simulink model "block_lms"  (Simulink 7.8)
settings: Solver=ode45  StartTime=0.0  StopTime=0.05  RelTol=1e-3
values from neighbouring files (symbols this model uses):
  h = firpm(64,f,m)    [CFIR_1.m]    (also in adapt_filter1.m = adaptfilt.lms(ni,mu); adapt_filter2.m = adaptfilt.blms(ni,mu,1,36); adaptiv_2.m = [1 2 3 4 5 6 7 8 9 10]; adaptiv_3.m = [1 2 3 4 5 6 7 8 9 10])
  hmusik = fir1(nf-1, 0.4)    [block_lms_.m]
  hr = 0.8.^(0:nf-1)    [block_lms_.m]
  M = 2    [CFIR_1.m]    (also in block_lms_.m = 16; cic_dezim1.m = ',num2str(M),'; cic_dezim1_.m = ',num2str(M),     '; cic_dezim2.m = ',num2str(M),')
  Ts = 1/fs    (= 6.25e-05)    [G722_1.m]    (also in adaptiv_2.m = 0.001; adaptiv_3.m = 0.001; adaptiv_4.m = 0.001; adaptiv_5.m = 0.001)
undefined symbols (not defined in the file or in its folder): get, stoerung
libraries: dspsigops x1, dspadpt3 x1, dspsrcs4 x1, dspsnks4 x1
settings Model: Creator=svenhoffmann  LastModifiedBy=josef  ExtModeAutoUpdateStatusClock=off
settings DataIOCC: SignalLoggingName=sigsOut
settings DebuggingCC: SaveWithParameterizedLinksMsg=none  SignalResolutionControl=TryResolveAllWithWarning  SolverPrmCheckMsg=none  MultiTaskDSMMsg=warning  MultiTaskCondExecSysMsg=none  StrictBusMsg=None
settings HardwareCC: TargetUnknown=on
settings RTWCC: IncludeERTFirstTime=on

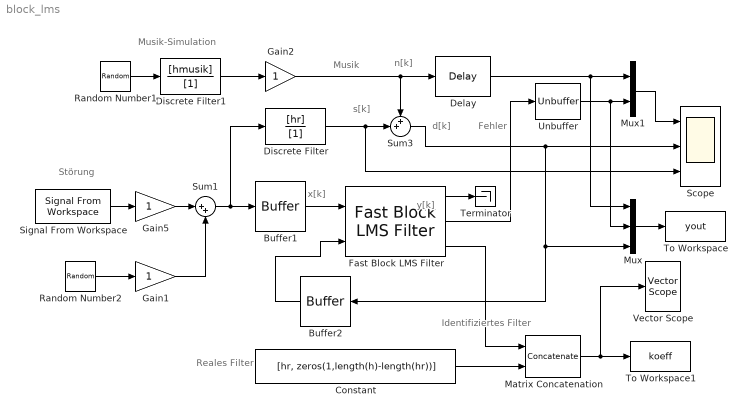
== system block_lms ==
  note: Musik
  note: Störung
  note: Musik-Simulation
  note: Fehler
  note: s[k]
  note: n[k]
  note: d[k]
  note: y[k]
  note: x[k]
  note: Reales Filter
  note: Identifiziertes Filter
  Buffer1 : Buffer  N=M
  Buffer2 : Buffer  N=M
  Constant : Constant  Value=[hr, zeros(1,length(h)-length(hr))]
  Delay : dspsigops/Delay  InputProcessing=Inherited (this choice will be removed - see release notes)  dly_unit=Samples  delay=M  ic_detail=off  dif_ic_for_ch=off  dif_ic_for_dly=off  ic=0  reset_popup=None
  Discrete Filter : DiscreteFilter  Numerator=[hr]  Denominator=[1]
  Discrete Filter1 : DiscreteFilter  Numerator=[hmusik]  Denominator=[1]  SampleTime=Ts
  Fast Block LMS Filter : dspadpt3/Fast Block LMS Filter  algo=Fast Block LMS  L=M  N=M  stepflag=Dialog  mu=0.002  leakage=1.0  addnparflag=off  ic=0  Adapt=off  resetflag=None  weights=on
  Gain1 : Gain  SaturateOnIntegerOverflow=on  OutDataTypeStr=Inherit: Same as input  ParamDataTypeStr=Inherit: Same as input
  Gain2 : Gain  SaturateOnIntegerOverflow=on  OutDataTypeStr=Inherit: Same as input  ParamDataTypeStr=Inherit: Same as input
  Gain5 : Gain  SaturateOnIntegerOverflow=on  OutDataTypeStr=Inherit: Same as input  ParamDataTypeStr=Inherit: Same as input
  Matrix Concatenation : Concatenate  Mode=Multidimensional array  ConcatenateDimension=2
  Mux : Mux  Inputs=3
  Mux1 : Mux  Inputs=2
  Random Number1 : RandomNumber  Seed=1739  SampleTime=Ts
  Random Number2 : RandomNumber  SampleTime=Ts
  Scope : Scope  NumInputPorts=3
      settings: YMin=-2.25~-2.25~-1  YMax=2.25~2.25~0.8
  Signal From Workspace : dspsrcs4/Signal From Workspace  X=stoerung(:,1)  Ts=Ts  nsamps=1  OutputAfterFinalValue=Setting to zero  ignoreOrWarnInputAndFrameLengths=off
  Sum1 : Sum  Inputs=|++  SaturateOnIntegerOverflow=on
  Sum3 : Sum  Inputs=++|  SaturateOnIntegerOverflow=on
  Terminator : Terminator
  To Workspace : ToWorkspace  VariableName=yout  SampleTime=-1  SaveFormat=Structure With Time
  To Workspace1 : ToWorkspace  VariableName=koeff  SampleTime=-1  SaveFormat=Structure
      settings: Decimation=100
  Unbuffer : Unbuffer
  Vector Scope : dspsnks4/Vector Scope  ScopeProperties=off  Domain=Time  HorizSpan=1  DisplayProperties=off  AxisGrid=on  Memory=off  FrameNumber=on  AxisLegend=off  AxisZoom=off  OpenScopeAtSimStart=on  OpenScopeImmediately=off  FigPos=get(0,'defaultfigureposition')  AxisProperties=off  XUnits=Hertz  XRange=[0...Fs/2]  InheritXIncr=on  XIncr=1  XLabel=Time  XLimit=Auto  XMin=0  XMax=1  XStart=0  YUnits=dB  YLabel=Amplitude  LineProperties=on  LineMarkers=*  XAxisParamsVer=6.8
      settings: YMin=-0.0150601797576505  YMax=1.05075300898788
  wires:
  Discrete Filter/1 -> Sum3/2, Scope/3
  Constant/1 -> Matrix Concatenation/2
  Matrix Concatenation/1 -> To Workspace1/1, Vector Scope/1
  Sum3/1 -> Scope/2, Mux/3, Buffer2/1
  Random Number1/1 -> Discrete Filter1/1
  Gain2/1 -> Sum3/1, Delay/1
  Discrete Filter1/1 -> Gain2/1
  Mux/1 -> To Workspace/1
  Fast Block LMS Filter/3 -> Matrix Concatenation/1
  Signal From Workspace/1 -> Gain5/1
  Mux1/1 -> Scope/1
  Gain5/1 -> Sum1/1
  Sum1/1 -> Discrete Filter/1, Buffer1/1
  Random Number2/1 -> Gain1/1
  Gain1/1 -> Sum1/2
  Buffer1/1 -> Fast Block LMS Filter/1
  Delay/1 -> Mux/1, Mux1/1
  Buffer2/1 -> Fast Block LMS Filter/2
  Unbuffer/1 -> Mux1/2, Mux/2
  Fast Block LMS Filter/1 -> Terminator/1
  Fast Block LMS Filter/2 -> Unbuffer/1
